simulink subsystem "Subsystem_Driver_BAv03"  (R2022b)
settings: Solver=VariableStepAuto  StartTime=0.0  StopTime=10.0  RelTol=1e-3
undefined symbols (not defined in the file): driver, route, weatherSim
settings Model: Creator=giaco  LastModifiedBy=giaco

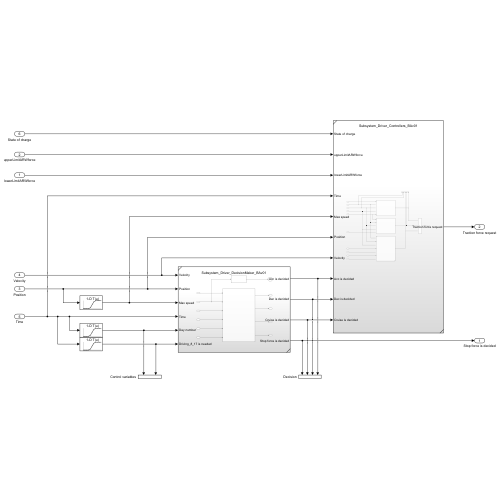
[thumbnail: Simulink's stored preview of the top-level diagram]
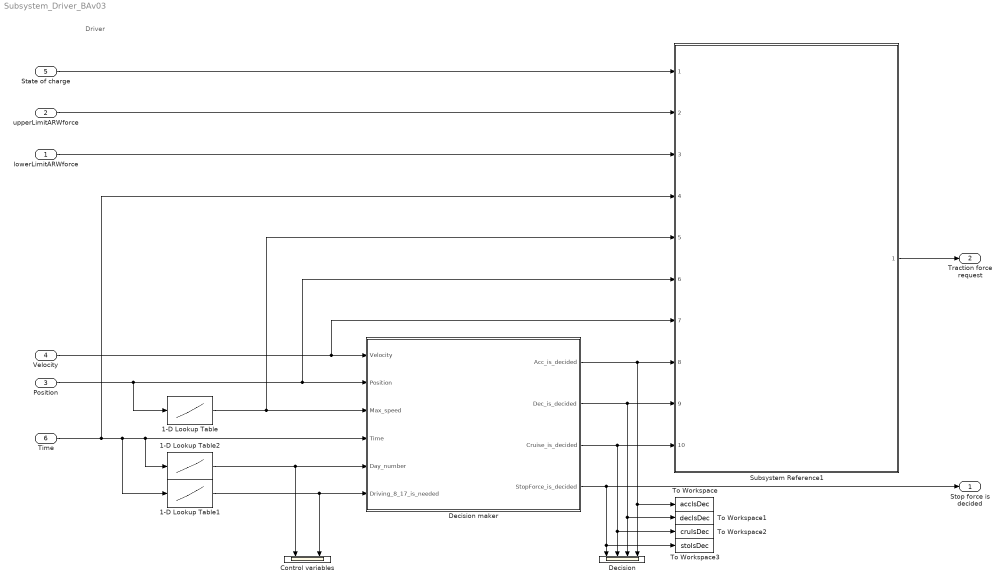
== system Subsystem_Driver_BAv03 ==
  note: Driver
  lowerLimitARWforce : Inport
  upperLimitARWforce : Inport  Port=2
  Position : Inport  Port=3
  Velocity : Inport  Port=4
  State of charge : Inport  Port=5
  Time : Inport  Port=6
  1-D Lookup Table : Lookup_n-D  NumberOfTableDimensions=1  BreakpointsForDimension1=route.dist  Table=route.maxSpeed  InternalRulePriority=Speed  RndMeth=Simplest
  1-D Lookup Table1 : Lookup_n-D  NumberOfTableDimensions=1  BreakpointsForDimension1=weatherSim.irradiance.timeSec  Table=weatherSim.irradiance.driving_8_17_Sec  InternalRulePriority=Speed
  1-D Lookup Table2 : Lookup_n-D  NumberOfTableDimensions=1  BreakpointsForDimension1=weatherSim.irradiance.timeSec  Table=weatherSim.irradiance.dayNumSec  InternalRulePriority=Speed
  Control variables : Scope  NumInputPorts=2
  Decision : Scope  NumInputPorts=4
  Decision maker : MATLAB Function  TreatAsAtomicUnit=on
  Subsystem Reference1 : Subsystem  ReferencedSubsystem=Subsystem_Driver_Controllers_BAv01
  To Workspace : ToWorkspace  VariableName=accIsDec  SaveFormat=Timeseries  SampleTime=-1
  To Workspace1 : ToWorkspace  VariableName=decIsDec  SaveFormat=Timeseries  SampleTime=-1
  To Workspace2 : ToWorkspace  VariableName=cruIsDec  SaveFormat=Timeseries  SampleTime=-1
  To Workspace3 : ToWorkspace  VariableName=stoIsDec  SaveFormat=Timeseries  SampleTime=-1
  Stop force is decided : Outport  OutDataTypeStr=boolean
  Traction force request : Outport  Port=2
  wires:
  Velocity/1 -> Decision maker/1(Velocity), Subsystem Reference1/7
  1-D Lookup Table1/1 -> Control variables/2, Decision maker/6(Driving_8_17_is_needed)
  State of charge/1 -> Subsystem Reference1/1
  Time/1 -> Subsystem Reference1/4, 1-D Lookup Table1/1, 1-D Lookup Table2/1, Decision maker/4(Time)
  Decision maker/4(StopForce_is_decided) -> Stop force is decided/1, Decision/1, To Workspace3/1
  1-D Lookup Table2/1 -> Decision maker/5(Day_number), Control variables/1
  1-D Lookup Table/1 -> Subsystem Reference1/5, Decision maker/3(Max_speed)
  Decision maker/3(Cruise_is_decided) -> Decision/2, To Workspace2/1, Subsystem Reference1/10
  Decision maker/2(Dec_is_decided) -> Decision/3, To Workspace1/1, Subsystem Reference1/9
  Decision maker/1(Acc_is_decided) -> Decision/4, To Workspace/1, Subsystem Reference1/8
  Subsystem Reference1/1 -> Traction force request/1
  upperLimitARWforce/1 -> Subsystem Reference1/2
  lowerLimitARWforce/1 -> Subsystem Reference1/3
  Position/1 -> 1-D Lookup Table/1, Decision maker/2(Position), Subsystem Reference1/6

== matlab function Subsystem_Driver_BAv03/Decision maker ==
  settings: updateMethod=DISCRETE
  data: Velocity input; Position input; Max_speed input; Time input; Day_number input; Driving_8_17_is_needed input; spaceStopIsOver data_store_memory; timeStopIsNeeded data_store_memory; spaceStopIsNeeded data_store_memory; driver parameter; spaceStopNumber data_store_memory; spaceStopIsStarted data_store_memory; Acc_is_decided output; Dec_is_decided output; Cruise_is_decided output; StopForce_is_decided output; spaceStopInitialTime data_store_memory; accInitialTime data_store_memory; accInitialVelocity data_store_memory; decInitialTime data_store_memory; decInitialVelocity data_store_memory; racingDayIsStarted data_store_memory; dayNumber data_store_memory; weatherSim parameter
function [Acc_is_decided, Dec_is_decided, Cruise_is_decided, StopForce_is_decided] = decisionMaker(Velocity, Position, Max_speed, Time, Day_number, Driving_8_17_is_needed, driver, weatherSim)

global racingDayIsStarted
global timeStopIsNeeded
global dayNumber

global spaceStopIsNeeded
global spaceStopIsStarted
global spaceStopIsOver
global spaceStopInitialTime
global spaceStopNumber

global accInitialTime
global accInitialVelocity
global decInitialTime
global decInitialVelocity

Acc_is_decided = false;
Dec_is_decided = false;
Cruise_is_decided = false;
StopForce_is_decided = false;

controlVelocity = min(driver.velRef, Max_speed);

%% Check for stops
% Time stops
stopTime = Time - Velocity ./ driver.decRef;

if ~timeStopIsNeeded && stopTime >= (weatherSim.irradiance.stopTimeSec(Day_number) - 60) %to be sure to stop on time
    timeStopIsNeeded = true;
    decInitialTime = Time; %initialization of time and velocity for ramp controller
    decInitialVelocity = Velocity;
end % if

% Space stops
stopDistance = Position - Velocity.^2 / (2 * driver.decRef);

if ~spaceStopIsNeeded && stopDistance >= driver.stopLocDist(spaceStopNumber)
    spaceStopIsNeeded = true;
    decInitialTime = Time; %initialization of time and velocity for ramp controller
    decInitialVelocity = Velocity;
    
    if spaceStopNumber < length(driver.stopLocDist) %omit last stop: stop simulation
        spaceStopNumber = spaceStopNumber + 1;
    end % if
end % if

%% Check for new racing day
if Driving_8_17_is_needed && Day_number == dayNumber
    racingDayIsStarted = true;
    timeStopIsNeeded = false;
    dayNumber = dayNumber + 1;
end % if

%% Select control options
%% Deceleration
if timeStopIsNeeded
    if Velocity > driver.velRefStop
        Dec_is_decided = true;
    else %if Velocity <= driver.velRefStop
        StopForce_is_decided = true;
        Dec_is_decided = false;
    end % if

elseif spaceStopIsNeeded
    if spaceStopIsStarted
        spaceStopDuration = Time - spaceStopInitialTime;
        if spaceStopDuration >= seconds(minutes(30))
            spaceStopIsNeeded = false;
            spaceStopIsStarted = false;
            spaceStopIsOver = true;
            Acc_is_decided = true;
            accInitialTime = Time;
            accInitialVelocity = Velocity;
        else
            StopForce_is_decided = true;
        end % if
    else
        if Velocity > driver.velRefStop
            Dec_is_decided = true;
        else %if Velocity < driver.velRefStop
            spaceStopIsStarted = true;
            spaceStopInitialTime = Time;
            StopForce_is_decided = true;
        end % if
    end % if

%% Acceleration
elseif racingDayIsStarted
    if Velocity < 0.9 * controlVelocity
        Acc_is_decided = true;
    else %if Velocity >= 0.9 * controlVelocity
        Cruise_is_decided = true;
        racingDayIsStarted = false;
    end % if

elseif spaceStopIsOver
    if Velocity < 0.9 * controlVelocity
        Acc_is_decided = true;
    else %if Velocity >= 0.9 * controlVelocity
        Cruise_is_decided = true;
        spaceStopIsOver = false;
    end % if

else
    Cruise_is_decided = true;
end % if
